simulink model "nasaBatterysim"  (R2019a)
settings: Solver=ode4  StartTime=0.0  StopTime=70  FixedStep=.01  RelTol=1e-3
settings Model: Creator=tdarrah  LastModifiedBy=tdarrah
settings DebuggingCC: ArithmeticOperatorsInVariantConditions=warning

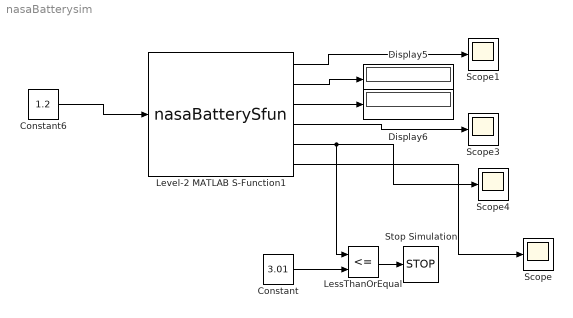
== system nasaBatterysim ==
  Constant : Constant  Value=3.01
  Constant6 : Constant  Value=1.2
  Display5 : Display
  Display6 : Display
  LessThanOrEqual : RelationalOperator  Operator=<=  OutDataTypeStr=boolean  RndMeth=Simplest
  Level-2 MATLAB S-Function1 : M-S-Function  FunctionName=nasaBatterySfun  Parameters=batteryParams
  Scope{,1,3..4} (4 alike) : Scope
  Stop Simulation : Stop
  wires:
  Level-2 MATLAB S-Function1/1 -> Scope1/1
  Level-2 MATLAB S-Function1/4 -> Scope3/1
  Level-2 MATLAB S-Function1/5 -> LessThanOrEqual/1, Scope4/1
  Level-2 MATLAB S-Function1/2 -> Display5/1
  Level-2 MATLAB S-Function1/3 -> Display6/1
  Constant6/1 -> Level-2 MATLAB S-Function1/1
  Constant/1 -> LessThanOrEqual/2
  LessThanOrEqual/1 -> Stop Simulation/1
  Level-2 MATLAB S-Function1/6 -> Scope/1
